simulink model "sf_demo_tl30"  (Simulink 7.8)
settings: Solver=FixedStepDiscrete  StartTime=0.0  StopTime=20  FixedStep=0.5  RelTol=1e-3
PreLoadFcn:
  | if exist('tl_preloadfcn','file'), tl_preloadfcn(gcs,101); end
PostLoadFcn:
  | if exist('tl_postloadfcn','file'), tl_postloadfcn(gcs,101); end
InitFcn:
  | if exist('tlds_init','file'), tlds_init(gcs); end
StartFcn:
  | if exist('tlds_start','file'), tlds_start(gcs); end
StopFcn:
  | if exist('tlds_stop','file'), tlds_stop(gcs); end
libraries: tllib x6
PreSaveFcn:
  | if exist('tl_presavefcn','file'), tl_presavefcn(gcs); end
settings Model: DS_PROJECTFILE=sf_demo_tl30.dd  TL_MAIN_DATA={'#advcodeopt',0,'codeopt',{'inliningthreshold',5,'assembler',1,'optlevel',0,'decimals',0},'frameopt',{'mexargs',''},'logopt',{'plotinterval',0.1,'globalloggingmode',4},'date',735046.66957627318}  TL_MODEL_COMMENT=This model implements a simple state machine.  TLRevision=101  Creator=rwilts  LastModifiedBy=Stefan  ExtModeTrigMode=oneshot  ExtModeArmWhenConnect=off  BufferReuse=off
settings DataIOCC: LimitDataPoints=off
settings OptimizationCC: BlockReduction=off  BooleanDataType=off  OptimizeBlockIOStorage=off  BufferReuse=off  ExpressionFolding=off  LocalBlockOutputs=off  InitFltsAndDblsToZero=on
settings DebuggingCC: SaveWithParameterizedLinksMsg=none  SignalResolutionControl=TryResolveAllWithWarning  SolverPrmCheckMsg=none  MultiTaskDSMMsg=warning  MultiTaskCondExecSysMsg=none  FcnCallInpInsideContextMsg=Use local settings
settings HardwareCC: TargetEndianess=LittleEndian  TargetHWDeviceType=MATLAB Host  ProdEqTarget=off
settings SFSimCC: SimParseCustomCode=off
settings RTWCC: IncludeERTFirstTime=on
settings GRTTargetCC: TargetFcnLib=ansi_tfl_tmw.mat

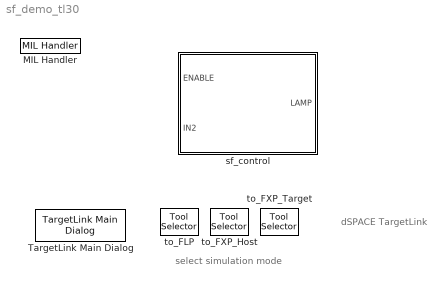
== system sf_demo_tl30 ==
  note: select simulation mode
  note: dSPACE TargetLink
  MIL Handler : tllib/MIL Handler  data={'date',735046.66957320599}
  TargetLink Main Dialog : tllib/TargetLink Main Dialog  data=[]
  sf_control : Subsystem  Tag=TargetLink Simulation Frame
      settings: CopyFcn=if exist('tl_copyfcn','file'), tl_copyfcn(gcbh); end  NameChangeFcn=if exist('tl_framenamechangefcn','file'), tl_framenamechangefcn(gcbh); end
      settings: OpenFcn=|
      | if exist('open_tlsubsystem','file')
      |    open_tlsubsystem(gcbh);
      | else
      |    tlsubsystem = ...
      |       find_system(gcb, ...
      |       'LookUnderMasks','on', ...
      |       'FollowLinks','on', ...
      |       'Tag','MIL Subsystem');
      |    open_system(tlsubsystem);
      | end
      mask Type: TL_SimFrame
      mask Display: disp('TargetLink\nModel-\nin-the-loop\nmode')
  to_FLP : tllib/Tool Selector  Description=MIL\nmode  data={'date',735046.66956687497}
  to_FXP_Host : tllib/Tool Selector  Description=SIL\nmode  data={'date',735046.66956668976}
  to_FXP_Target : tllib/Tool Selector  Description=PIL\nmode  data={'date',735046.66956668976}

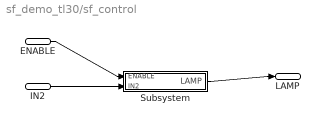
== system sf_demo_tl30/sf_control ==
  ENABLE : Inport  OutDataTypeStr=osc_int16  SampleTime=0.5  LockScale=on
  IN2 : Inport  Port=2  OutDataTypeStr=osc_int16  SampleTime=0.5
  Subsystem : Subsystem  Tag=struct('sfcnName','sf_control_sf','subFunction','','srcSubsystem','')
      settings: OpenFcn=warndlg(get_param(gcb,'MaskHelp'),'Serious Warning');
      mask Type: TL_Enable
      mask Help: This subsystem keeps the TargetLink subsystem (subsystem with TargetLink blocks for production code generation), and is needed for the TargetLink simulation frame to work properly. DO NOT DELETE OR MODIFY IT!
  LAMP : Outport
  wires:
  ENABLE/1 -> Subsystem/1(ENABLE)
  IN2/1 -> Subsystem/2(IN2)
  Subsystem/1(LAMP) -> LAMP/1

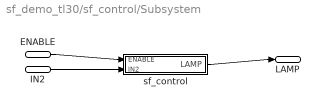
== system sf_demo_tl30/sf_control/Subsystem ==
  ENABLE : Inport  OutDataTypeStr=osc_int16  SampleTime=0.5
  IN2 : Inport  Port=2  OutDataTypeStr=osc_int16  SampleTime=0.5
  sf_control : Subsystem  Tag=MIL Subsystem  Description=a
      settings: CopyFcn=if exist('tl_copyfcn','file'), tl_copyfcn(gcbh); end  NameChangeFcn=if exist('tl_namechangefcn','file'), tl_namechangefcn(gcbh); end  DestroyFcn=if exist('update_tl_main_dlg','file'), update_tl_main_dlg('TL_subs_display'); end
      mask Display: disp('TargetLink Subsystem')
  LAMP : Outport
  wires:
  ENABLE/1 -> sf_control/1(ENABLE)
  IN2/1 -> sf_control/2(IN2)
  sf_control/1(LAMP) -> LAMP/1

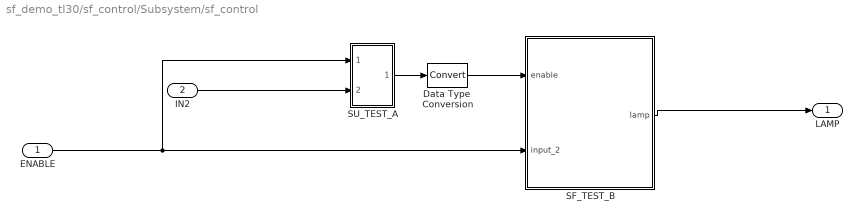
== system sf_demo_tl30/sf_control/Subsystem/sf_control ==
  ENABLE : Inport  OutDataTypeStr=osc_int16  PortDimensions=1  SampleTime=0.5  mask(TL_Inport){data={'logdata',{'maxnumvals',4096,'plotchannels',1,'loggingmode',1},'output',{'max',1,'min',0,'class','FCN_ARG','type','Int8'},'date',735046.66957302089}}
      settings: DeleteFcn=if exist('delete_tlblock','file')==2,delete_tlblock(gcbh);end  OpenFcn=if exist('tl_open_blockdlg','file')==2,tl_open_blockdlg(gcbh);else,open_system(gcbh,'parameter');end
      settings: CopyFcn=|
      | if exist('tl_reset_reviewflag','file')==2
      |     tl_reset_reviewflag(gcbh);
      | end
      | if exist('tl_check_ports','file')
      |     tl_check_ports(gcbh);
      | end
      settings: NameChangeFcn=|
      | if exist('rename_tlblock','file')==2,rename_tlblock(gcbh);end
      | if exist('tl_check_ports','file'), tl_check_ports(gcbh); end
      mask Help: eval(['if exist(''tl_online_help'',''file'') == 2, tl_online_help(''Topic'',''TL_Inport''),else, web([''jar:file:///'',matlabroot,''/help/toolbox/simulink/help.jar!/slref/' lower(get_param(gcbh,'Blocktype')) '.html''], ''-helpbrowser''),end'])
      mask Display: plot([0.2 0.35 NaN 0.65 0.8],[0 1 NaN 0 1]);
  IN2 : Inport  Port=2  OutDataTypeStr=osc_int16  PortDimensions=1  SampleTime=0.5  mask(TL_Inport){data={'logdata',{'maxnumvals',4096,'plotchannels',1,'loggingmode',1},'output',{'max',1,'min',0,'class','FCN_ARG','type','Int8'},'date',735046.66957211809}}
      settings: DeleteFcn=if exist('delete_tlblock','file')==2,delete_tlblock(gcbh);end  OpenFcn=if exist('tl_open_blockdlg','file')==2,tl_open_blockdlg(gcbh);else,open_system(gcbh,'parameter');end
      settings: CopyFcn=|
      | if exist('tl_reset_reviewflag','file')==2
      |     tl_reset_reviewflag(gcbh);
      | end
      | if exist('tl_check_ports','file')
      |     tl_check_ports(gcbh);
      | end
      settings: NameChangeFcn=|
      | if exist('rename_tlblock','file')==2,rename_tlblock(gcbh);end
      | if exist('tl_check_ports','file'), tl_check_ports(gcbh); end
      mask Help: eval(['if exist(''tl_online_help'',''file'') == 2, tl_online_help(''Topic'',''TL_Inport''),else, web([''jar:file:///'',matlabroot,''/help/toolbox/simulink/help.jar!/slref/' lower(get_param(gcbh,'Blocktype')) '.html''], ''-helpbrowser''),end'])
      mask Display: plot([0.2 0.35 NaN 0.65 0.8],[0 1 NaN 0 1]);
  Data Type  Conversion : DataTypeConversion  SaturateOnIntegerOverflow=on  RndMeth=Zero
  SF_TEST_B : Stateflow chart  TreatAsAtomicUnit=on
  SU_TEST_A : Subsystem  TreatAsAtomicUnit=on
  LAMP : Outport  OutDataTypeStr=int32  PortDimensions=1  mask(TL_Outport){data={'logdata',{'plotchannels',1},'output',{'max',1,'min',0,'class','DISP','type','UInt8'},'autoscaling',{'mode',2},'date',735046.66956741898}}
      settings: DeleteFcn=if exist('delete_tlblock','file')==2,delete_tlblock(gcbh);end  OpenFcn=if exist('tl_open_blockdlg','file')==2,tl_open_blockdlg(gcbh);else,open_system(gcbh,'parameter');end
      settings: CopyFcn=|
      | if exist('tl_reset_reviewflag','file')==2
      |     tl_reset_reviewflag(gcbh);
      | end
      | if exist('tl_check_ports','file')
      |     tl_check_ports(gcbh);
      | end
      settings: NameChangeFcn=|
      | if exist('rename_tlblock','file')==2,rename_tlblock(gcbh);end
      | if exist('tl_check_ports','file'), tl_check_ports(gcbh); end
      mask Help: eval(['if exist(''tl_online_help'',''file'') == 2, tl_online_help(''Topic'',''TL_Outport''),else, web([''jar:file:///'',matlabroot,''/help/toolbox/simulink/help.jar!/slref/' lower(get_param(gcbh,'Blocktype')) '.html''], ''-helpbrowser''),end'])
      mask Display: plot([0.2 0.35 NaN 0.65 0.8],[0 1 NaN 0 1]);
  wires:
  SF_TEST_B/1(lamp) -> LAMP/1
  ENABLE/1 -> SU_TEST_A/1(In1), SF_TEST_B/2(input_2)
  IN2/1 -> SU_TEST_A/2(In2)
  SU_TEST_A/1(Out1) -> Data Type  Conversion/1
  Data Type  Conversion/1 -> SF_TEST_B/1(enable)

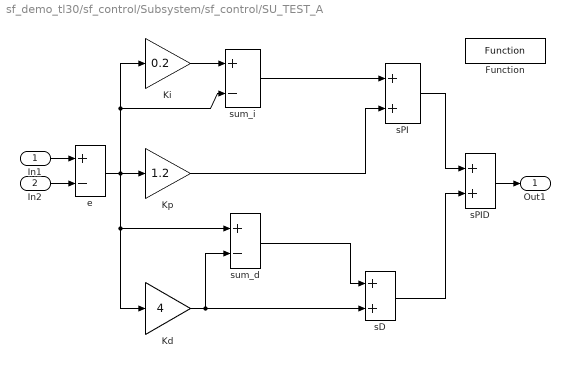
== system sf_demo_tl30/sf_control/Subsystem/sf_control/SU_TEST_A ==
  In1 : Inport  OutDataTypeStr=osc_int16
  In2 : Inport  Port=2  OutDataTypeStr=osc_int16
  Function : tllib/Function  data={'date',735046.66956650466}
  Kd : Gain  Tag="Gain block of the dSPACE Fixed Point Code Generation Environment.      \\n                                                                       \\n signal is equal to the product of the input signal and the gain value:\\n\t\ty = G u"  Description=|  Gain=4  OutDataTypeStr=Inherit: Inherit via back propagation  mask(TL_Gain){data={'logdata',{'plotchannels',1},'output',{'type','Int8','lsb',2^-15},'gain',{'name','P_$D','class','CAL','type','UInt8','lsb',2^-5},'date',735046.66957121529}}
      | Gain block of dSPACE TargetLink.
      | 
      | Output signal is equal to the product of the input signal and the gain value:
      |         y = G u
      settings: CopyFcn=if exist('tl_reset_reviewflag','file')==2,tl_reset_reviewflag(gcbh);end  DeleteFcn=if exist('delete_tlblock','file')==2,delete_tlblock(gcbh);end  NameChangeFcn=if exist('rename_tlblock','file')==2,rename_tlblock(gcbh);end  OpenFcn=if exist('tl_open_blockdlg','file')==2,tl_open_blockdlg(gcbh);else,open_system(gcbh,'parameter');end
      mask Help: eval(['if exist(''tl_online_help'',''file'') == 2, tl_online_help(''Topic'',''TL_Gain''),else, web([''jar:file:///'',matlabroot,''/help/toolbox/simulink/help.jar!/slref/' lower(get_param(gcbh,'Blocktype')) '.html''], ''-helpbrowser''),end'])
      mask Display: plot([0, .9, 0],[.05, .5, .95])
  Ki : Gain  Description=|  Gain=0.2  mask(TL_Gain){data={'logdata',{'plotchannels',[]},'output',{'lsb',2^-20},'gain',{'name','P_$D','class','CAL','type','UInt8','lsb',2^-10},'date',735046.66957084485}}
      | Gain block of dSPACE TargetLink.
      | 
      | Output signal is equal to the product of the input signal and the gain value:
      |         y = G u
      settings: CopyFcn=if exist('tl_reset_reviewflag','file')==2,tl_reset_reviewflag(gcbh);end  DeleteFcn=if exist('delete_tlblock','file')==2,delete_tlblock(gcbh);end  NameChangeFcn=if exist('rename_tlblock','file')==2,rename_tlblock(gcbh);end  OpenFcn=if exist('tl_open_blockdlg','file')==2,tl_open_blockdlg(gcbh);else,open_system(gcbh,'parameter');end
      mask Help: eval(['if exist(''tl_online_help'',''file'') == 2, tl_online_help(''Topic'',''TL_Gain''),else, web([''jar:file:///'',matlabroot,''/help/toolbox/simulink/help.jar!/slref/' lower(get_param(gcbh,'Blocktype')) '.html''], ''-helpbrowser''),end'])
      mask Display: plot([0, .9, 0],[.05, .5, .95])
  Kp : Gain  Tag="Gain block of the dSPACE Fixed Point Code Generation Environment.      \\n                                                                       \\n signal is equal to the product of the input signal and the gain value:\\n\t\ty = G u"  Description=|  Gain=1.2  mask(TL_Gain){data={'logdata',{'plotchannels',[]},'output',{'lsb',2^-17},'gain',{'name','P_$D','class','CAL','type','UInt8','lsb',2^-7},'date',735046.66957031249}}
      | Gain block of dSPACE TargetLink.
      | 
      | Output signal is equal to the product of the input signal and the gain value:
      |         y = G u
      settings: CopyFcn=if exist('tl_reset_reviewflag','file')==2,tl_reset_reviewflag(gcbh);end  DeleteFcn=if exist('delete_tlblock','file')==2,delete_tlblock(gcbh);end  NameChangeFcn=if exist('rename_tlblock','file')==2,rename_tlblock(gcbh);end  OpenFcn=if exist('tl_open_blockdlg','file')==2,tl_open_blockdlg(gcbh);else,open_system(gcbh,'parameter');end
      mask Help: eval(['if exist(''tl_online_help'',''file'') == 2, tl_online_help(''Topic'',''TL_Gain''),else, web([''jar:file:///'',matlabroot,''/help/toolbox/simulink/help.jar!/slref/' lower(get_param(gcbh,'Blocktype')) '.html''], ''-helpbrowser''),end'])
      mask Display: plot([0, .9, 0],[.05, .5, .95])
  e : Sum  Description=|  Inputs=+-  mask(TL_Sum){data={'logdata',{'plotchannels',1,'loggingmode',1},'output',{'lsb',2^-18,'checkmin',1,'checkmax',1},'date',735046.66956976848}}
      | Sum block of dSPACE TargetLink.
      | 
      | Output signal is equal to the sum of the input signals.
      | The list of signs is specified according to conventions for Simulink Sum blocks.
      settings: CopyFcn=if exist('tl_reset_reviewflag','file')==2,tl_reset_reviewflag(gcbh);end  DeleteFcn=if exist('delete_tlblock','file')==2,delete_tlblock(gcbh);end  NameChangeFcn=if exist('rename_tlblock','file')==2,rename_tlblock(gcbh);end  OpenFcn=if exist('tl_open_blockdlg','file')==2,tl_open_blockdlg(gcbh);else,open_system(gcbh,'parameter');end
      mask Help: eval(['if exist(''tl_online_help'',''file'') == 2, tl_online_help(''Topic'',''TL_Sum''),else, web([''jar:file:///'',matlabroot,''/help/toolbox/simulink/help.jar!/slref/' lower(get_param(gcbh,'Blocktype')) '.html''], ''-helpbrowser''),end'])
      mask Display: plot([-0.05, 1.05, NaN, -0.05, 1.05],[.01, .01, NaN, .99, .99])
  sD : Sum  Tag="Sum block of the dSPACE Fixed Point Code Generation Environment.\\n                                                                \\nOutput signal is equal to the sum of the two input signals:     \\n                                                                \\n\t\ty = u1 - u2"  Description=|  OutDataTypeStr=Inherit: Inherit via back propagation  mask(TL_Sum){data={'logdata',{'plotchannels',1},'output',{'lsb',2^-15},'date',735046.66956939816}}
      | Sum block of dSPACE TargetLink.
      | 
      | Output signal is equal to the sum of the input signals.
      | The list of signs is specified according to conventions for Simulink Sum blocks.
      settings: CopyFcn=if exist('tl_reset_reviewflag','file')==2,tl_reset_reviewflag(gcbh);end  DeleteFcn=if exist('delete_tlblock','file')==2,delete_tlblock(gcbh);end  NameChangeFcn=if exist('rename_tlblock','file')==2,rename_tlblock(gcbh);end  OpenFcn=if exist('tl_open_blockdlg','file')==2,tl_open_blockdlg(gcbh);else,open_system(gcbh,'parameter');end
      mask Help: eval(['if exist(''tl_online_help'',''file'') == 2, tl_online_help(''Topic'',''TL_Sum''),else, web([''jar:file:///'',matlabroot,''/help/toolbox/simulink/help.jar!/slref/' lower(get_param(gcbh,'Blocktype')) '.html''], ''-helpbrowser''),end'])
      mask Display: plot([-0.05, 1.05, NaN, -0.05, 1.05],[.01, .01, NaN, .99, .99])
  sPI : Sum  Tag="Sum block of the dSPACE Fixed Point Code Generation Environment.\\n                                                                \\nOutput signal is equal to the sum of the two input signals:     \\n                                                                \\n\t\ty = u1 - u2"  Description=|  OutDataTypeStr=Inherit: Inherit via back propagation  mask(TL_Sum){data={'logdata',{'plotchannels',[]},'output',{'lsb',2^-17},'date',735046.66956903937}}
      | Sum block of dSPACE TargetLink.
      | 
      | Output signal is equal to the sum of the input signals.
      | The list of signs is specified according to conventions for Simulink Sum blocks.
      settings: CopyFcn=if exist('tl_reset_reviewflag','file')==2,tl_reset_reviewflag(gcbh);end  DeleteFcn=if exist('delete_tlblock','file')==2,delete_tlblock(gcbh);end  NameChangeFcn=if exist('rename_tlblock','file')==2,rename_tlblock(gcbh);end  OpenFcn=if exist('tl_open_blockdlg','file')==2,tl_open_blockdlg(gcbh);else,open_system(gcbh,'parameter');end
      mask Help: eval(['if exist(''tl_online_help'',''file'') == 2, tl_online_help(''Topic'',''TL_Sum''),else, web([''jar:file:///'',matlabroot,''/help/toolbox/simulink/help.jar!/slref/' lower(get_param(gcbh,'Blocktype')) '.html''], ''-helpbrowser''),end'])
      mask Display: plot([-0.05, 1.05, NaN, -0.05, 1.05],[.01, .01, NaN, .99, .99])
  sPID : Sum  Description=|  OutDataTypeStr=Inherit: Inherit via back propagation  mask(TL_Sum){data={'logdata',{'plotchannels',1},'output',{'lsb',2^-15},'date',735046.66956868058}}
      | Sum block of dSPACE TargetLink.
      | 
      | Output signal is equal to the sum of the input signals.
      | The list of signs is specified according to conventions for Simulink Sum blocks.
      settings: CopyFcn=if exist('tl_reset_reviewflag','file')==2,tl_reset_reviewflag(gcbh);end  DeleteFcn=if exist('delete_tlblock','file')==2,delete_tlblock(gcbh);end  NameChangeFcn=if exist('rename_tlblock','file')==2,rename_tlblock(gcbh);end  OpenFcn=if exist('tl_open_blockdlg','file')==2,tl_open_blockdlg(gcbh);else,open_system(gcbh,'parameter');end
      mask Help: eval(['if exist(''tl_online_help'',''file'') == 2, tl_online_help(''Topic'',''TL_Sum''),else, web([''jar:file:///'',matlabroot,''/help/toolbox/simulink/help.jar!/slref/' lower(get_param(gcbh,'Blocktype')) '.html''], ''-helpbrowser''),end'])
      mask Display: plot([-0.05, 1.05, NaN, -0.05, 1.05],[.01, .01, NaN, .99, .99])
  sum_d : Sum  Description=|  Inputs=+-  OutDataTypeStr=Inherit: Inherit via back propagation  mask(TL_Sum){data={'logdata',{'plotchannels',[]},'output',{'lsb',2^-15},'date',735046.66956832178}}
      | Sum block of dSPACE TargetLink.
      | 
      | Output signal is equal to the sum of the input signals.
      | The list of signs is specified according to conventions for Simulink Sum blocks.
      settings: CopyFcn=if exist('tl_reset_reviewflag','file')==2,tl_reset_reviewflag(gcbh);end  DeleteFcn=if exist('delete_tlblock','file')==2,delete_tlblock(gcbh);end  NameChangeFcn=if exist('rename_tlblock','file')==2,rename_tlblock(gcbh);end  OpenFcn=if exist('tl_open_blockdlg','file')==2,tl_open_blockdlg(gcbh);else,open_system(gcbh,'parameter');end
      mask Help: eval(['if exist(''tl_online_help'',''file'') == 2, tl_online_help(''Topic'',''TL_Sum''),else, web([''jar:file:///'',matlabroot,''/help/toolbox/simulink/help.jar!/slref/' lower(get_param(gcbh,'Blocktype')) '.html''], ''-helpbrowser''),end'])
      mask Display: plot([-0.05, 1.05, NaN, -0.05, 1.05],[.01, .01, NaN, .99, .99])
  sum_i : Sum  Tag="Sum block of the dSPACE Fixed Point Code Generation Environment.\\n                                                                \\nOutput signal is equal to the sum of the two input signals:     \\n                                                                \\n\t\ty = u1 - u2"  Description=|  Inputs=+-  mask(TL_Sum){data={'logdata',{'plotchannels',[]},'output',{'lsb',2^-19},'date',735046.66956795135}}
      | Sum block of dSPACE TargetLink.
      | 
      | Output signal is equal to the sum of the input signals.
      | The list of signs is specified according to conventions for Simulink Sum blocks.
      settings: CopyFcn=if exist('tl_reset_reviewflag','file')==2,tl_reset_reviewflag(gcbh);end  DeleteFcn=if exist('delete_tlblock','file')==2,delete_tlblock(gcbh);end  NameChangeFcn=if exist('rename_tlblock','file')==2,rename_tlblock(gcbh);end  OpenFcn=if exist('tl_open_blockdlg','file')==2,tl_open_blockdlg(gcbh);else,open_system(gcbh,'parameter');end
      mask Help: eval(['if exist(''tl_online_help'',''file'') == 2, tl_online_help(''Topic'',''TL_Sum''),else, web([''jar:file:///'',matlabroot,''/help/toolbox/simulink/help.jar!/slref/' lower(get_param(gcbh,'Blocktype')) '.html''], ''-helpbrowser''),end'])
      mask Display: plot([-0.05, 1.05, NaN, -0.05, 1.05],[.01, .01, NaN, .99, .99])
  Out1 : Outport
  wires:
  Kd/1 -> sum_d/2, sD/2
  sD/1 -> sPID/2
  sum_d/1 -> sD/1
  sPI/1 -> sPID/1
  sum_i/1 -> sPI/1
  Ki/1 -> sum_i/1
  Kp/1 -> sPI/2
  e/1 -> Kp/1, Ki/1, sum_i/2, Kd/1, sum_d/1
  In1/1 -> e/1
  In2/1 -> e/2
  sPID/1 -> Out1/1

== stateflow chart sf_control/Subsystem/sf_control/SF_TEST_B ==
  settings: sampleTime=1
  state do_blink
    state BLINKER_ON/
      entry:lamp=1;
    state BLINKER_OFF
      entry: lamp = 0;
    BLINKER_ON -> BLINKER_OFF
    BLINKER_OFF -> BLINKER_ON
  state OFF
    entry: lamp = 0;
  (default) -> OFF
  OFF -> BLINKER_ON : [enable == 1]
  do_blink -> OFF : [enable==0]
  data: enable input osc_boolean; lamp output osc_int32; input_2 input osc_int16
  data enable settings: description=$TL$ createinputvariable=1; $TL$
  data input_2 settings: description=$TL$ createinputvariable=1; $TL$
